simulink model "simulinkFIRDA"  (R2020b)
settings: Solver=VariableStepAuto  StartTime=0.0  StopTime=100  RelTol=1e-3
undefined symbols (not defined in the file): magnitude
libraries: simulink x3
settings Model: Creator=admin  LastModifiedBy=firda
settings SolverCC: ZeroCrossAlgorithm=Adaptive  AlgebraicLoopSolver=LineSearch
settings DataIOCC: ReturnWorkspaceOutputs=off
settings DebuggingCC: MaskedZcDiagnostic=none  IgnoredZcDiagnostic=none  ArithmeticOperatorsInVariantConditions=warning
settings SFSimCC: SimUseLocalCustomCode=off  CustomCodeUndefinedFunction=UseInterfaceOnly
settings RTWCC: RTWUseLocalCustomCode=off
settings CodeAppCC: StateflowObjectComments=on

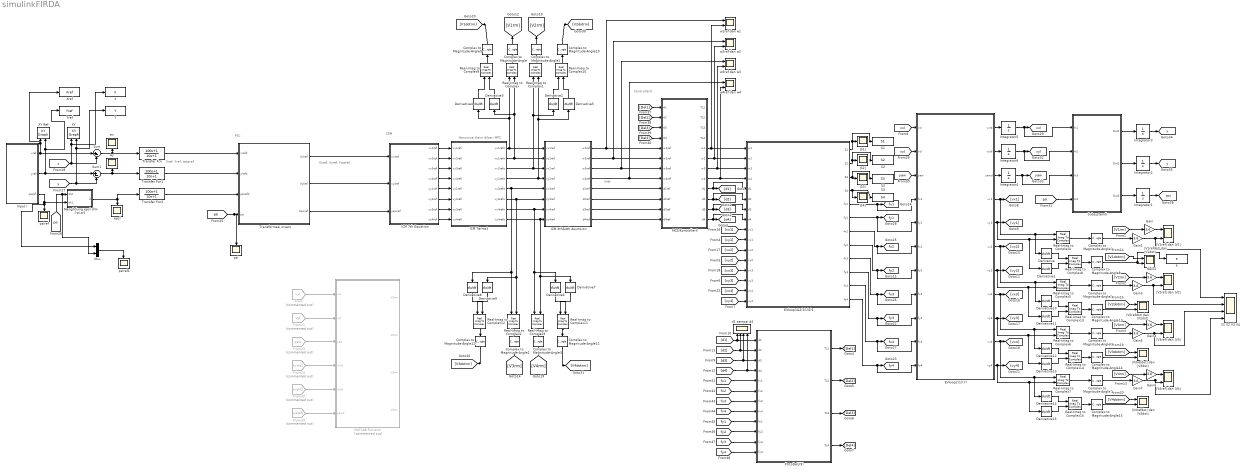
== system simulinkFIRDA ==
  note: Harusnya disini diberi MPC
  note: ControllerX
  note: C8M
  note: Xref, Yref, tetaref
  note: PTC
  note: Vxref, Vyref, Yawref
  note: Xref
  Complex to Magnitude-Angle{,1..15} (16 alike) : ComplexToMagnitudeAngle  Output=Magnitude
  Derivative{,1..15} (16 alike) : Derivative
  EVloop1&2(3)-(6)1 : Subsystem  mask(Vehicle body dinamic){re1=0.32, re2=0.32, re3=0.32, re4=0.32, m=1000, g=9.8, h=0.42, ld=0.75, lf=1.42, lr=1.42, kro=20972, kfo=50539, ksj=0.95}
      mask prompts: re1 "jari-jari roda 1 (m)"; re2 "jari-jari roda 2 (m)"; re3 "jari-jari roda 3 (m)"; re4 "jari-jari roda 4 (m)"; m "massa kendaraan (kg)"; g "percepatan gravitasi (m/s^2)"; h "tinggi pusat massa dari permukaan jalan (m)"; ld "jarak pusat massa ke bodi samping (m)"; lf "jarak pusat massa ke bodi depan (m)"; lr "jarak pusat massa ke bodi belakang (m)"; kro "ketegangan roll belakang"; kfo "ketegangan roll depan"; ksj "faktor atenuasi"
      mask help: Persamaan (3)(4)(5)(6)
  EVloop2(1)(7) : Subsystem  mask(Vehicle bodi dinamic){m=1000, ld=0.75, lf=1.42, lr=1.42, Jz=1950}
      mask prompts: m "massa kendaraan (kg)"; ld "jarak pusat massa ke bodi samping (m)"; lf "jarak pusat massa ke bodi depan (m)"; lr "jarak pusat massa ke bodi belakang (m)"; Jz "the moment of inertia of the vehicle about an axis through its CM"
      mask help: Loop 2 Persamaan 1 & 7
  From : From  Commented=on  GotoTag=vxl  TagVisibility=global
  From21 : From  Commented=on  GotoTag=vyl  TagVisibility=global
  From23 : From  Commented=on  GotoTag=yaw  TagVisibility=global
  From24 : From  Commented=on  GotoTag=vxld
  From32 : From  Commented=on  GotoTag=vyld
  From33 : From  Commented=on  GotoTag=yawd
  FtrtoDelj(9) : Subsystem  mask(Vehicle body dinamic){jm1=0.36, jm2=0.36, jm3=0.36, jm4=0.36, re1=0.32, re2=0.32, re3=0.32, re4=0.32}
      mask prompts: jm1 "momen inersia roda 1 (kgm^2)"; jm2 "momen inersia roda 2 (kgm^2)"; jm3 "momen inersia roda 3 (kgm^2)"; jm4 "momen inersia roda 4 (kgm^2)"; re1 "jari-jari roda 1 (m)"; re2 "jari-jari roda 2 (m)"; re3 "jari-jari roda 3 (m)"; re4 "jari-jari roda 4 (m)"
      mask help: Persamaan (9)
  Gain{,1..7} (8 alike) : Gain  Gain=3.6
  ICM 3th&4th Asumsion : Subsystem  mask(Persamaan ICM){rej=0.32}
      mask prompts: rej "Jari-jari roda (m)"
      mask help:
      | Asumsi 3 (Zero Slip), bidang roda berhimpit dengan Vj, aj=0,
      | djref=sudut apit (vxjref dan vyjref)
      | Asumsi 4 (Free Rolling), slip longitudinal SLj=0,
      | wjref= norm(vxjref,vyjref)/rej
  ICM 7th Equation : Subsystem  mask(Persamaan ICM){ld=0.75, lf=1.42, lr=1.42}
      mask prompts: ld "Jarak pusat masa ke bodi samping (m)"; lf "Jarak pusat masa ke bodi depan (m)"; lr "Jarak pusat masa ke bodi belakang (m)"
      mask help:
      | mengkoordinasikan kecepatan masing-masing roda
      | terhadap kecepatan pusat kendaraan
      | dengan menggunakan konsep ICM
  ICM Terms1 : Subsystem  mask(Ketentuan ICM){}
      mask help:
      | djref tidak terdefinisi ketika vxjref=vyjref=0
      | vxjref dan vyjref mengambil nilai sebelumnya saat keduanya sama dengan nol
  Input r : Subsystem  mask{Ts=0.01}
      mask prompts: Ts "Sample Period"
      mask Display: image('D:\icon mask\eight curved.jpg');
  Integrator{1..4,6} (5 alike) : Integrator
  Integrator5 : Integrator  InitialCondition=1.6
  MATLAB Function : MATLAB Function  Commented=on  TreatAsAtomicUnit=on  mask{Ts=0.01, Nc=2, Np=10, t=100, Qmat=0, Rmat=0}
      mask prompts: Ts "Sampling Time"; Nc "Control Horizon (Nc)"; Np "Prediction Horizon (Np)"; t "Run Time"; Qmat "Q"; Rmat "R"
  MCS/KontrollerX : Subsystem  mask(MCS/Kontroller X){}
      mask help: Melacak nilai torsi dan ws dari Xref
  Menghtiung epsi dlm [-pi,pi] : MATLAB Function  TreatAsAtomicUnit=on
  Mux : Mux  Inputs=2
  Real-Imag to Complex{,1..15} (16 alike) : RealImagToComplex
  S1 : ToWorkspace  VariableName=S1  SampleTime=-1
      settings: Save2DSignal=2-D array (concatenate along first dimension)
  S2 : ToWorkspace  VariableName=S2  SampleTime=-1
      settings: Save2DSignal=2-D array (concatenate along first dimension)
  S3 : ToWorkspace  VariableName=S3  SampleTime=-1
      settings: Save2DSignal=2-D array (concatenate along first dimension)
  S4 : ToWorkspace  VariableName=S4  SampleTime=-1
      settings: Save2DSignal=2-D array (concatenate along first dimension)
  Subsystem5 : Subsystem
  Sum : Sum  Inputs=|+-
  Sum1 : Sum  Inputs=|+-
  Transfer Fcn : TransferFcn  Numerator=[100 1]  Denominator=[10 1]
  Transfer Fcn1 : TransferFcn  Numerator=[100 1]  Denominator=[10 1]
  Transfer Fcn2 : TransferFcn  Numerator=[100 1]  Denominator=[10 1]
  "Transformasi invers " : Subsystem  mask(Tranformasi){}
      mask help: Mengubah Xdot menjadi Vxl Vyl Yaw
      mask Display: image('D:\icon mask\transformasi.jpg');
  V1 V2 V3 V4 : Scope  NumInputPorts=4
  X : ToWorkspace  VariableName=X  SampleTime=-1
      settings: Save2DSignal=2-D array (concatenate along first dimension)
  "XY " : simulink/Sinks/XY Graph  xmin=-40  xmax=200  ymin=-5  ymax=85  st=0.5
  XY Ref : simulink/Sinks/XY Graph  xmin=-40  xmax=200  ymin=-5  ymax=85  st=0.5
  Xref : ToWorkspace  VariableName=Xref  SampleTime=-1
      settings: Save2DSignal=2-D array (concatenate along first dimension)
  Y : ToWorkspace  VariableName=Y  SampleTime=-1
      settings: Save2DSignal=2-D array (concatenate along first dimension)
  Yref : ToWorkspace  VariableName=Yref  SampleTime=-1
      settings: Save2DSignal=2-D array (concatenate along first dimension)
  a : ToWorkspace  VariableName=a  SampleTime=-1
      settings: Save2DSignal=2-D array (concatenate along first dimension)
  d1 sampai d4 : Scope  NumInputPorts=4
  epsi : Scope
  ex : Scope
  ey : Scope
  psi : Scope
  psiref : Scope
  psiref1 : Scope
  w1ref dan w1 : Scope  NumInputPorts=2
  w2ref dan w2 : Scope  NumInputPorts=2
  w3ref dan w3 : Scope  NumInputPorts=2
  w4ref dan w4 : Scope  NumInputPorts=2
  |S1| : Scope
  |S2| : Scope
  |S3| : Scope
  |S4| : Scope
  |V1refdot| dan |V1dot| : Scope  NumInputPorts=2
  |V1ref| dan |V1| : Scope  NumInputPorts=2
  |V2refdot| dan |V2dot| : Scope  NumInputPorts=2
  |V2ref| dan |V2| : Scope  NumInputPorts=2
  |V3refdot| dan |V3dot| : Scope  NumInputPorts=2
  |V3ref| dan |V3| : Scope  NumInputPorts=2
  |V4refdot| dan |V4dot| : Scope  NumInputPorts=2
  |V4ref| dan |V4| : Scope  NumInputPorts=2
  tag scope: fx1=global, fx2=global, fx3=global, fx4=global, fy1=global, fy2=global, fy3=global, fy4=global, psi=global, vxl=global, vyl=global, x=global, y=global, yaw=global
  wires:
  [x] -> Sum/2, X/1, "XY "/1
  [y] -> Sum1/2, Y/1, "XY "/2
  [vx4] -> EVloop1&2(3)-(6)1/15(vx4)
  [vx3] -> EVloop1&2(3)-(6)1/13(vx3)
  Transfer Fcn1/1 -> "Transformasi invers "/2(yrefd)
  Transfer Fcn2/1 -> "Transformasi invers "/3(psirefd)
  "Transformasi invers "/1(Vxlref) -> ICM 7th Equation/1(vxlref)
  "Transformasi invers "/2(Vylref) -> ICM 7th Equation/2(vylref)
  "Transformasi invers "/3(Yawref) -> ICM 7th Equation/3(yawref)
  EVloop1&2(3)-(6)1/12(fy4) -> EVloop2(1)(7)/11(fy4), [fy4]
  EVloop1&2(3)-(6)1/10(fy3) -> EVloop2(1)(7)/9(fy3), [fy3]
  EVloop1&2(3)-(6)1/5(fx1) -> EVloop2(1)(7)/4(fx1), [fx1]
  EVloop1&2(3)-(6)1/7(fx2) -> EVloop2(1)(7)/6(fx2), [fx2]
  EVloop1&2(3)-(6)1/8(fy2) -> EVloop2(1)(7)/7(fy2), [fy2]
  EVloop1&2(3)-(6)1/6(fy1) -> EVloop2(1)(7)/5(fy1), [fy1]
  [vy4] -> EVloop1&2(3)-(6)1/16(vy4)
  [vy3] -> EVloop1&2(3)-(6)1/14(vy3)
  [vy2] -> EVloop1&2(3)-(6)1/12(vy2)
  [vx2] -> EVloop1&2(3)-(6)1/11(vx2)
  [vy1] -> EVloop1&2(3)-(6)1/10(vy1)
  [vx1] -> EVloop1&2(3)-(6)1/9(vx1)
  [Del1] -> MCS/KontrollerX/1(tl1)
  [Del2] -> MCS/KontrollerX/2(tl2)
  ICM 3th&4th Asumsion/1(w1ref) -> MCS/KontrollerX/5(w1ref), w1ref dan w1/1
  ICM 3th&4th Asumsion/5(d1ref) -> MCS/KontrollerX/9(d1ref)
  ICM 3th&4th Asumsion/2(w2ref) -> MCS/KontrollerX/6(w2ref), w2ref dan w2/1
  [Del3] -> MCS/KontrollerX/3(tl3)
  ICM 3th&4th Asumsion/6(d2ref) -> MCS/KontrollerX/10(d2ref)
  ICM 3th&4th Asumsion/3(w3ref) -> MCS/KontrollerX/7(w3ref), w3ref dan w3/1
  ICM 3th&4th Asumsion/7(d3ref) -> MCS/KontrollerX/11(d3ref)
  [Del4] -> MCS/KontrollerX/4(tl4)
  ICM 3th&4th Asumsion/4(w4ref) -> MCS/KontrollerX/8(w4ref), w4ref dan w4/1
  ICM 3th&4th Asumsion/8(d4ref) -> MCS/KontrollerX/12(d4ref)
  Integrator3/1 -> [x]
  Integrator2/1 -> [y]
  Integrator1/1 -> [psi]
  EVloop1&2(3)-(6)1/9(fx3) -> EVloop2(1)(7)/8(fx3), [fx3]
  EVloop1&2(3)-(6)1/11(fx4) -> EVloop2(1)(7)/10(fx4), [fx4]
  [vxl] -> EVloop2(1)(7)/1(vxl)
  [vyl] -> EVloop2(1)(7)/2(vyl)
  [yaw] -> EVloop2(1)(7)/3(yaw)
  EVloop2(1)(7)/4(vx1) -> Derivative/1, Real-Imag to Complex4/1, [vx1]
  EVloop2(1)(7)/5(vy1) -> Derivative1/1, Real-Imag to Complex4/2, [vy1]
  EVloop2(1)(7)/1(vxld) -> Integrator5/1
  Integrator5/1 -> Subsystem5/1(In1), [vxl]
  EVloop2(1)(7)/2(vyld) -> Integrator6/1
  Integrator6/1 -> Subsystem5/2(In2), [vyl]
  EVloop2(1)(7)/3(yawd) -> Integrator4/1
  Integrator4/1 -> Subsystem5/3(In3), [yaw]
  [psi] -> Subsystem5/4(In4)
  Subsystem5/1(Out1) -> Integrator3/1
  Subsystem5/2(Out2) -> Integrator2/1
  Subsystem5/3(Out3) -> Integrator1/1
  MCS/KontrollerX/9(d1) -> EVloop1&2(3)-(6)1/5(d1), [d1]
  MCS/KontrollerX/10(d2) -> EVloop1&2(3)-(6)1/6(d2), [d2]
  MCS/KontrollerX/11(d3) -> EVloop1&2(3)-(6)1/7(d3), [d3]
  MCS/KontrollerX/12(d4) -> EVloop1&2(3)-(6)1/8(d4), [d4]
  MCS/KontrollerX/5(w1) -> EVloop1&2(3)-(6)1/1(w1), w1ref dan w1/2
  MCS/KontrollerX/6(w2) -> EVloop1&2(3)-(6)1/2(w2), w2ref dan w2/2
  MCS/KontrollerX/7(w3) -> EVloop1&2(3)-(6)1/3(w3), w3ref dan w3/2
  MCS/KontrollerX/8(w4) -> EVloop1&2(3)-(6)1/4(w4), w4ref dan w4/2
  Transfer Fcn/1 -> "Transformasi invers "/1(xrefd)
  ICM 7th Equation/1(vx1ref) -> ICM Terms1/1(vx1refi)
  ICM 7th Equation/2(vx2ref) -> ICM Terms1/2(vx2refi)
  ICM 7th Equation/3(vx3ref) -> ICM Terms1/3(vx3refi)
  ICM 7th Equation/4(vx4ref) -> ICM Terms1/4(vx4refi)
  ICM 7th Equation/5(vy1ref) -> ICM Terms1/5(vy1refi)
  ICM 7th Equation/6(vy2ref) -> ICM Terms1/6(vy2refi)
  ICM 7th Equation/7(vy3ref) -> ICM Terms1/7(vy3refi)
  ICM 7th Equation/8(vy4ref) -> ICM Terms1/8(vy4refi)
  ICM Terms1/1(vx1refo) -> ICM 3th&4th Asumsion/1(vx1ref), Derivative4/1, Real-Imag to Complex/1
  ICM Terms1/2(vy1refo) -> ICM 3th&4th Asumsion/2(vy1ref), Derivative3/1, Real-Imag to Complex/2
  ICM Terms1/3(vx2refo) -> Real-Imag to Complex1/1, Derivative2/1, ICM 3th&4th Asumsion/3(vx2ref)
  ICM Terms1/4(vy2refo) -> Derivative5/1, Real-Imag to Complex1/2, ICM 3th&4th Asumsion/4(vy2ref)
  Sum/1 -> Transfer Fcn/1, ex/1
  Sum1/1 -> ey/1, Transfer Fcn1/1
  Input r/1(xref) -> Sum/1, Xref/1, XY Ref/1
  EVloop1&2(3)-(6)1/1(S1) -> S1/1, |S1|/1
  Input r/2(yref) -> Sum1/1, Yref/1, XY Ref/2
  EVloop1&2(3)-(6)1/2(S2) -> S2/1, |S2|/1
  EVloop1&2(3)-(6)1/3(S3) -> |S3|/1, S3/1
  EVloop1&2(3)-(6)1/4(S4) -> |S4|/1, S4/1
  [fy3] -> FtrtoDelj(9)/11(fy3)
  [fy1] -> FtrtoDelj(9)/9(fy1)
  [d1] -> FtrtoDelj(9)/1(d1), d1 sampai d4/1
  FtrtoDelj(9)/3(TL3) -> [Del3]
  [fy2] -> FtrtoDelj(9)/10(fy2)
  FtrtoDelj(9)/1(TL1) -> [Del1]
  FtrtoDelj(9)/2(TL2) -> [Del2]
  [d3] -> FtrtoDelj(9)/3(d3), d1 sampai d4/3
  [d4] -> d1 sampai d4/4, FtrtoDelj(9)/4(d4)
  [fx4] -> FtrtoDelj(9)/8(fx4)
  [fx1] -> FtrtoDelj(9)/5(fx1)
  [fx3] -> FtrtoDelj(9)/7(fx3)
  [d2] -> FtrtoDelj(9)/2(d2), d1 sampai d4/2
  [fx2] -> FtrtoDelj(9)/6(fx2)
  [fy4] -> FtrtoDelj(9)/12(fy4)
  FtrtoDelj(9)/4(TL4) -> [Del4]
  Real-Imag to Complex/1 -> Complex to Magnitude-Angle/1
  Complex to Magnitude-Angle/1 -> [V1rm]
  Real-Imag to Complex1/1 -> Complex to Magnitude-Angle1/1
  Complex to Magnitude-Angle1/1 -> [V2rm]
  Real-Imag to Complex2/1 -> Complex to Magnitude-Angle2/1
  Complex to Magnitude-Angle2/1 -> [V3rm]
  Complex to Magnitude-Angle3/1 -> [V4rm]
  Real-Imag to Complex3/1 -> Complex to Magnitude-Angle3/1
  Real-Imag to Complex4/1 -> Complex to Magnitude-Angle4/1
  Complex to Magnitude-Angle4/1 -> Gain1/1
  Real-Imag to Complex5/1 -> Complex to Magnitude-Angle5/1
  Complex to Magnitude-Angle5/1 -> Gain3/1
  [V2rm] -> Gain2/1
  Real-Imag to Complex6/1 -> Complex to Magnitude-Angle6/1
  Complex to Magnitude-Angle6/1 -> Gain5/1
  [V3rm] -> Gain4/1
  Real-Imag to Complex7/1 -> Complex to Magnitude-Angle7/1
  [V4rm] -> Gain6/1
  [psi] -> psi/1, "Transformasi invers "/4(psi)
  Input r/3("psiref ") -> Menghtiung epsi dlm [-pi,pi]/2(th1), Mux/1, psiref/1
  [psi] -> Mux/2, Menghtiung epsi dlm [-pi,pi]/1(th2)
  Menghtiung epsi dlm [-pi,pi]/1(d) -> Transfer Fcn2/1, epsi/1
  Derivative/1 -> Real-Imag to Complex8/1
  Derivative1/1 -> Real-Imag to Complex8/2
  Real-Imag to Complex8/1 -> Complex to Magnitude-Angle8/1
  Derivative3/1 -> Real-Imag to Complex9/2
  Derivative4/1 -> Real-Imag to Complex9/1
  Complex to Magnitude-Angle9/1 -> [V1dotrm]
  Real-Imag to Complex9/1 -> Complex to Magnitude-Angle9/1
  Complex to Magnitude-Angle10/1 -> [V2dotrm]
  Derivative5/1 -> Real-Imag to Complex10/2
  Derivative2/1 -> Real-Imag to Complex10/1
  Real-Imag to Complex10/1 -> Complex to Magnitude-Angle10/1
  Complex to Magnitude-Angle11/1 -> [V4dotrm]
  Derivative6/1 -> Real-Imag to Complex11/2
  ICM Terms1/7(vx4refo) -> ICM 3th&4th Asumsion/7(vx4ref), Derivative6/1, Real-Imag to Complex3/1
  ICM Terms1/8(vy4refo) -> ICM 3th&4th Asumsion/8(vy4ref), Derivative7/1, Real-Imag to Complex3/2
  Derivative7/1 -> Real-Imag to Complex11/1
  Real-Imag to Complex11/1 -> Complex to Magnitude-Angle11/1
  Complex to Magnitude-Angle12/1 -> [V3dotrm]
  Derivative8/1 -> Real-Imag to Complex12/2
  ICM Terms1/5(vx3refo) -> ICM 3th&4th Asumsion/5(vx3ref), Real-Imag to Complex2/1, Derivative8/1
  ICM Terms1/6(vy3refo) -> ICM 3th&4th Asumsion/6(vy3ref), Real-Imag to Complex2/2, Derivative9/1
  Derivative9/1 -> Real-Imag to Complex12/1
  Real-Imag to Complex12/1 -> Complex to Magnitude-Angle12/1
  [V2dotrm] -> |V2refdot| dan |V2dot|/1
  EVloop2(1)(7)/7(vy2) -> Derivative11/1, Real-Imag to Complex5/2, [vy2]
  Derivative10/1 -> Real-Imag to Complex13/1
  Complex to Magnitude-Angle13/1 -> |V2refdot| dan |V2dot|/2
  Real-Imag to Complex13/1 -> Complex to Magnitude-Angle13/1
  Derivative11/1 -> Real-Imag to Complex13/2
  EVloop2(1)(7)/6(vx2) -> Derivative10/1, Real-Imag to Complex5/1, [vx2]
  [V3dotrm] -> |V3refdot| dan |V3dot|/1
  EVloop2(1)(7)/9(vy3) -> Derivative13/1, Real-Imag to Complex6/2, [vy3]
  Derivative12/1 -> Real-Imag to Complex14/1
  Complex to Magnitude-Angle14/1 -> |V3refdot| dan |V3dot|/2
  Real-Imag to Complex14/1 -> Complex to Magnitude-Angle14/1
  Derivative13/1 -> Real-Imag to Complex14/2
  EVloop2(1)(7)/8(vx3) -> Derivative12/1, Real-Imag to Complex6/1, [vx3]
  [V4dotrm] -> |V4refdot| dan |V4dot|/1
  EVloop2(1)(7)/11(vy4) -> Derivative15/1, Real-Imag to Complex7/2, [vy4]
  Derivative14/1 -> Real-Imag to Complex15/1
  Complex to Magnitude-Angle15/1 -> |V4refdot| dan |V4dot|/2
  Real-Imag to Complex15/1 -> Complex to Magnitude-Angle15/1
  Derivative15/1 -> Real-Imag to Complex15/2
  EVloop2(1)(7)/10(vx4) -> Derivative14/1, Real-Imag to Complex7/1, [vx4]
  Complex to Magnitude-Angle7/1 -> Gain7/1
  [V1rm] -> Gain/1
  Gain/1 -> |V1ref| dan |V1|/1
  Gain1/1 -> V1 V2 V3 V4/1, |V1ref| dan |V1|/2
  Gain2/1 -> |V2ref| dan |V2|/1
  Gain3/1 -> V1 V2 V3 V4/2, |V2ref| dan |V2|/2
  Gain4/1 -> |V3ref| dan |V3|/1
  Gain5/1 -> |V3ref| dan |V3|/2, V1 V2 V3 V4/3
  Gain6/1 -> |V4ref| dan |V4|/1
  Gain7/1 -> V1 V2 V3 V4/4, |V4ref| dan |V4|/2
  Complex to Magnitude-Angle8/1 -> a/1, |V1refdot| dan |V1dot|/2
  Mux/1 -> psiref1/1
  From/1 -> MATLAB Function/1(vxl)
  From21/1 -> MATLAB Function/2(vyl)
  From23/1 -> MATLAB Function/3(yaw)
  From33/1 -> MATLAB Function/6(yawd)
  From32/1 -> MATLAB Function/5(vyld)
  From24/1 -> MATLAB Function/4(vxld)
  [V1dotrm] -> |V1refdot| dan |V1dot|/1

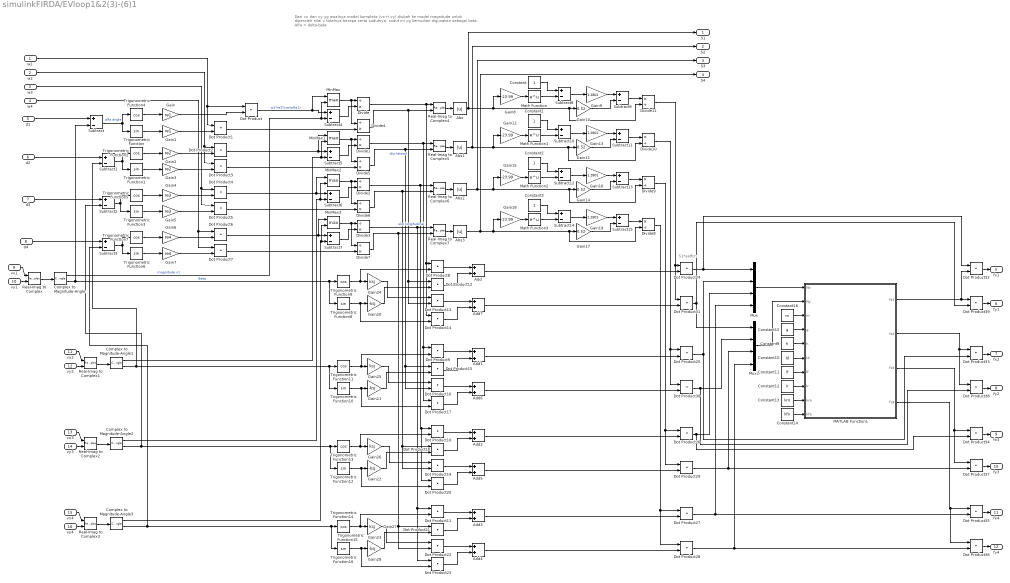
== system simulinkFIRDA/EVloop1&2(3)-(6)1 ==
  note: S1*satfcn
  note: Dari vx dan vy yg awalnya model kompleks (vx+i vy) diubah ke model magnitude untuk diperoleh nilai v totalnya berapa serta sudutnya. sudut ini yg kemudian digunakan sebagai beta.
      | Alfa = delta-beta
  w1 : Inport
  w2 : Inport  Port=2
  w3 : Inport  Port=3
  w4 : Inport  Port=4
  d1 : Inport  Port=5
  d2 : Inport  Port=6
  d3 : Inport  Port=7
  d4 : Inport  Port=8
  vx1 : Inport  Port=9
  vy1 : Inport  Port=10
  vx2 : Inport  Port=11
  vy2 : Inport  Port=12
  vx3 : Inport  Port=13
  vy3 : Inport  Port=14
  vx4 : Inport  Port=15
  vy4 : Inport  Port=16
  Abs{,1..3} (4 alike) : Abs
  Add{,1..7} (8 alike) : Sum
  Complex to Magnitude-Angle{,1..3} (4 alike) : ComplexToMagnitudeAngle
  Constant{,1..3} (4 alike) : Constant
  Constant10 : Constant  Value=ld
  Constant11 : Constant  Value=lf
  Constant12 : Constant  Value=lr
  Constant13 : Constant  Value=kro
  Constant14 : Constant  Value=kfo
  Constant15 : Constant  Value=g
  Constant16 : Constant  Value=m
  Constant9 : Constant  Value=h
  Divide{,1..7} (8 alike) : Product  Inputs=/*
  Divide{8..11} (4 alike) : Product  Inputs=*/
  Dot Product{,1..39} (40 alike) : DotProduct  InputSameDT=on  OutDataTypeStr=Inherit: Inherit via internal rule
  Gain : Gain  Gain=re1
  Gain1 : Gain  Gain=re1
  Gain{10..11,14,17} (4 alike) : Gain  Gain=0.52
  Gain{8,12,15,18} (4 alike) : Gain  Gain=-23.99
  Gain{9,13,16,19} (4 alike) : Gain  Gain=1.2801
  Gain2 : Gain  Gain=re2
  Gain{20..23,28} (5 alike) : Gain  Gain=-ksj
  Gain{24..27} (4 alike) : Gain  Gain=ksj
  Gain3 : Gain  Gain=re2
  Gain4 : Gain  Gain=re3
  Gain5 : Gain  Gain=re3
  Gain6 : Gain  Gain=re4
  Gain7 : Gain  Gain=re4
  MATLAB Function1 : MATLAB Function  TreatAsAtomicUnit=on
  Math Function{,1..3} (4 alike) : Math  SignedPower=on  SaturateOnIntegerOverflow=on
  MinMax{,1..3} (4 alike) : MinMax  Function=max  Inputs=2
  Mux : Mux
  Mux1 : Mux
  Real-Imag to Complex{,1..7} (8 alike) : RealImagToComplex
  Subtract{,1..15} (16 alike) : Sum  Inputs=+-
  Trigonometric Function{,1,3,6,8,10,12,14,16} (9 alike) : Trigonometry
  Trigonometric Function{2,4..5,7,9,11,13,15} (8 alike) : Trigonometry  Operator=cos
  S1 : Outport
  S2 : Outport  Port=2
  S3 : Outport  Port=3
  S4 : Outport  Port=4
  fx1 : Outport  Port=5
  fy1 : Outport  Port=6
  fx2 : Outport  Port=7
  fy2 : Outport  Port=8
  fx3 : Outport  Port=9
  fy3 : Outport  Port=10
  fx4 : Outport  Port=11
  fy4 : Outport  Port=12
  wires:
  Dot Product33/1 -> fx2/1
  Dot Product35/1 -> fx4/1
  Dot Product28/1 -> Dot Product36/2, Mux1/4
  Dot Product36/1 -> fy4/1
  Dot Product34/1 -> fx3/1
  Dot Product39/1 -> fy1/1
  Dot Product37/1 -> fy3/1
  Dot Product38/1 -> fy2/1
  Dot Product32/1 -> fx1/1
  vx1/1 -> Real-Imag to Complex/1
  vy1/1 -> Real-Imag to Complex/2
  vx3/1 -> Real-Imag to Complex2/1
  vy3/1 -> Real-Imag to Complex2/2
  vx4/1 -> Real-Imag to Complex3/1
  vx2/1 -> Real-Imag to Complex1/1
  vy4/1 -> Real-Imag to Complex3/2
  vy2/1 -> Real-Imag to Complex1/2
  Constant15/1 -> MATLAB Function1/4(g)
  Dot Product31/1 -> Dot Product39/2, Mux1/1
  Dot Product29/1 -> Dot Product37/2, Mux1/3
  Dot Product30/1 -> Dot Product38/2, Mux1/2
  Constant16/1 -> MATLAB Function1/3(m)
  MATLAB Function1/1(fz1) -> Dot Product32/2, Dot Product39/1
  MATLAB Function1/3(fz3) -> Dot Product34/1, Dot Product37/1
  Constant14/1 -> MATLAB Function1/10(kfo)
  Constant13/1 -> MATLAB Function1/9(kro)
  Real-Imag to Complex2/1 -> Complex to Magnitude-Angle2/1
  Real-Imag to Complex3/1 -> Complex to Magnitude-Angle3/1
  Complex to Magnitude-Angle/2 -> Trigonometric Function8/1, Trigonometric Function9/1, Subtract/2  "Beta"
  Complex to Magnitude-Angle1/2 -> Trigonometric Function10/1, Trigonometric Function11/1, Subtract1/2
  Real-Imag to Complex/1 -> Complex to Magnitude-Angle/1
  Real-Imag to Complex1/1 -> Complex to Magnitude-Angle1/1
  Trigonometric Function1/1 -> Gain3/1
  w1/1 -> Dot Product1/1, Dot Product/1
  Trigonometric Function5/1 -> Gain4/1
  d4/1 -> Subtract3/1
  Subtract/1 -> Trigonometric Function/1, Trigonometric Function4/1  "alfa angle"
  Gain4/1 -> Dot Product4/2
  w2/1 -> Dot Product2/1, Dot Product3/1
  w4/1 -> Dot Product6/1, Dot Product7/1
  Subtract2/1 -> Trigonometric Function3/1, Trigonometric Function5/1
  d3/1 -> Subtract2/1
  Gain5/1 -> Dot Product5/2
  Gain/1 -> Dot Product/2
  Dot Product2/1 -> MinMax1/1, Subtract5/1
  Gain1/1 -> Dot Product1/2
  d1/1 -> Subtract/1
  Gain3/1 -> Dot Product3/2
  Gain7/1 -> Dot Product7/2
  Trigonometric Function6/1 -> Gain7/1
  Dot Product/1 -> Subtract4/1, MinMax/1  "w1*re1*cos(alfa1)"
  Complex to Magnitude-Angle3/2 -> Subtract3/2, Trigonometric Function16/1, Trigonometric Function14/1, Trigonometric Function15/1
  Trigonometric Function4/1 -> Gain/1
  Complex to Magnitude-Angle2/2 -> Trigonometric Function12/1, Trigonometric Function13/1, Subtract2/2
  Subtract1/1 -> Trigonometric Function2/1, Trigonometric Function1/1
  Trigonometric Function2/1 -> Gain2/1
  Trigonometric Function3/1 -> Gain5/1
  Gain6/1 -> Dot Product6/2
  Trigonometric Function/1 -> Gain1/1
  Gain2/1 -> Dot Product2/2
  w3/1 -> Dot Product4/1, Dot Product5/1
  Trigonometric Function7/1 -> Gain6/1
  d2/1 -> Subtract1/1
  Subtract3/1 -> Trigonometric Function6/1, Trigonometric Function7/1
  Complex to Magnitude-Angle/1 -> MinMax/2, Subtract4/2  "magnitude v1"
  Real-Imag to Complex5/1 -> Abs1/1
  Divide3/1 -> Dot Product23/1, Dot Product11/1, Real-Imag to Complex7/1
  Dot Product5/1 -> Divide6/2
  Divide/1 -> Dot Product14/1, Dot Product8/1, Real-Imag to Complex4/1  "slip longitudinal"
  Real-Imag to Complex6/1 -> Abs2/1
  MinMax3/1 -> Divide7/1, Divide3/1
  Divide7/1 -> Dot Product22/2, Dot Product21/1, Real-Imag to Complex7/2
  MinMax1/1 -> Divide5/1, Divide1/1
  Dot Product3/1 -> Divide5/2
  Dot Product7/1 -> Divide7/2
  Subtract5/1 -> Divide1/2
  Divide6/1 -> Dot Product19/2, Dot Product18/1, Real-Imag to Complex6/2
  Real-Imag to Complex7/1 -> Abs3/1
  Complex to Magnitude-Angle3/1 -> MinMax3/2, Subtract7/2
  Dot Product4/1 -> MinMax2/1, Subtract6/1
  Dot Product6/1 -> MinMax3/1, Subtract7/1
  Real-Imag to Complex4/1 -> Abs/1
  Gain8/1 -> Math Function/1
  Subtract6/1 -> Divide2/2
  Math Function/1 -> Subtract8/2
  Divide4/1 -> Dot Product13/2, Dot Product12/1, Real-Imag to Complex4/2  "slip lateral"
  Complex to Magnitude-Angle2/1 -> MinMax2/2, Subtract6/2
  Dot Product1/1 -> Divide4/2
  Subtract4/1 -> Divide/2
  Complex to Magnitude-Angle1/1 -> MinMax1/2, Subtract5/2
  MinMax/1 -> Divide4/1, Divide/1
  Subtract7/1 -> Divide3/2
  Divide5/1 -> Dot Product15/1, Dot Product16/2, Real-Imag to Complex5/2
  Divide2/1 -> Dot Product20/1, Dot Product10/1, Real-Imag to Complex6/1
  MinMax2/1 -> Divide6/1, Divide2/1
  Divide1/1 -> Dot Product9/1, Dot Product17/1, Real-Imag to Complex5/1
  Gain9/1 -> Subtract9/1
  Gain12/1 -> Math Function1/1
  Trigonometric Function8/1 -> Dot Product14/2, Gain20/1
  Trigonometric Function10/1 -> Dot Product17/2, Gain21/1
  Gain10/1 -> Subtract9/2
  Subtract8/1 -> Gain9/1
  Trigonometric Function14/1 -> Gain23/1
  Subtract14/1 -> Gain19/1
  Abs3/1 -> S4/1, Gain18/1, Gain17/1, Divide8/2
  Abs2/1 -> S3/1, Gain15/1, Divide9/2, Gain14/1
  Subtract13/1 -> Divide9/1
  Subtract10/1 -> Gain13/1
  Gain18/1 -> Math Function3/1
  Subtract15/1 -> Divide8/1
  Constant2/1 -> Subtract12/1
  Constant1/1 -> Subtract10/1
  Constant3/1 -> Subtract14/1
  Trigonometric Function12/1 -> Dot Product20/2, Gain22/1
  Abs1/1 -> S2/1, Gain12/1, Divide10/2, Gain11/1
  Trigonometric Function9/1 -> Dot Product8/2, Gain24/1
  Gain16/1 -> Subtract13/1
  Gain17/1 -> Subtract15/2
  Constant/1 -> Subtract8/1
  Math Function1/1 -> Subtract10/2
  Gain13/1 -> Subtract11/1
  Math Function2/1 -> Subtract12/2
  Subtract12/1 -> Gain16/1
  Gain15/1 -> Math Function2/1
  Gain14/1 -> Subtract13/2
  Math Function3/1 -> Subtract14/2
  Gain19/1 -> Subtract15/1
  Gain11/1 -> Subtract11/2
  Divide9/1 -> Dot Product26/1, Dot Product29/1
  Dot Product11/1 -> Add3/1
  Trigonometric Function13/1 -> Dot Product10/2, Gain26/1
  Add3/1 -> Dot Product27/2
  Dot Product10/1 -> Add2/1
  Add2/1 -> Dot Product26/2
  Dot Product21/1 -> Add3/2
  Divide8/1 -> Dot Product28/1, Dot Product27/1
  Trigonometric Function16/1 -> Dot Product23/2, Gain28/1
  Gain24/1 -> Dot Product13/1
  Dot Product9/1 -> Add1/1
  Gain25/1 -> Dot Product16/1
  Gain26/1 -> Dot Product19/1
  Gain27/1 -> Dot Product22/1
  Add4/1 -> Dot Product28/2
  Divide11/1 -> Dot Product31/1, Dot Product24/1
  Dot Product18/1 -> Add2/2
  Add/1 -> Dot Product24/2
  Gain20/1 -> Dot Product12/2
  Dot Product8/1 -> Add/1
  Gain21/1 -> Dot Product15/2
  Gain22/1 -> Dot Product18/2
  Dot Product15/1 -> Add1/2
  Divide10/1 -> Dot Product30/1, Dot Product25/1
  Abs/1 -> S1/1, Gain8/1, Divide11/2, Gain10/1
  Trigonometric Function11/1 -> Dot Product9/2, Gain25/1
  Gain28/1 -> Dot Product21/2
  Trigonometric Function15/1 -> Dot Product11/2, Gain27/1
  Subtract9/1 -> Divide11/1
  Add1/1 -> Dot Product25/2
  Dot Product12/1 -> Add/2
  Subtract11/1 -> Divide10/1
  Add7/1 -> Dot Product31/2
  Dot Product22/1 -> Add4/1
  Dot Product16/1 -> Add6/1
  Add5/1 -> Dot Product29/2
  Dot Product17/1 -> Add6/2
  Dot Product13/1 -> Add7/1
  Dot Product19/1 -> Add5/1
  Dot Product14/1 -> Add7/2
  Add6/1 -> Dot Product30/2
  Dot Product23/1 -> Add4/2
  Dot Product20/1 -> Add5/2
  Dot Product27/1 -> Dot Product35/2, Mux/4
  Constant11/1 -> MATLAB Function1/7(lf)
  Dot Product25/1 -> Dot Product33/2, Mux/2
  Constant9/1 -> MATLAB Function1/5(h)
  Dot Product24/1 -> Dot Product32/1, Mux/1
  Constant10/1 -> MATLAB Function1/6(ld)
  Mux1/1 -> MATLAB Function1/2(Ny)
  Constant12/1 -> MATLAB Function1/8(lr)
  MATLAB Function1/4(fz4) -> Dot Product36/1, Dot Product35/1
  MATLAB Function1/2(fz2) -> Dot Product33/1, Dot Product38/1
  Dot Product26/1 -> Dot Product34/2, Mux/3
  Mux/1 -> MATLAB Function1/1(Nx)

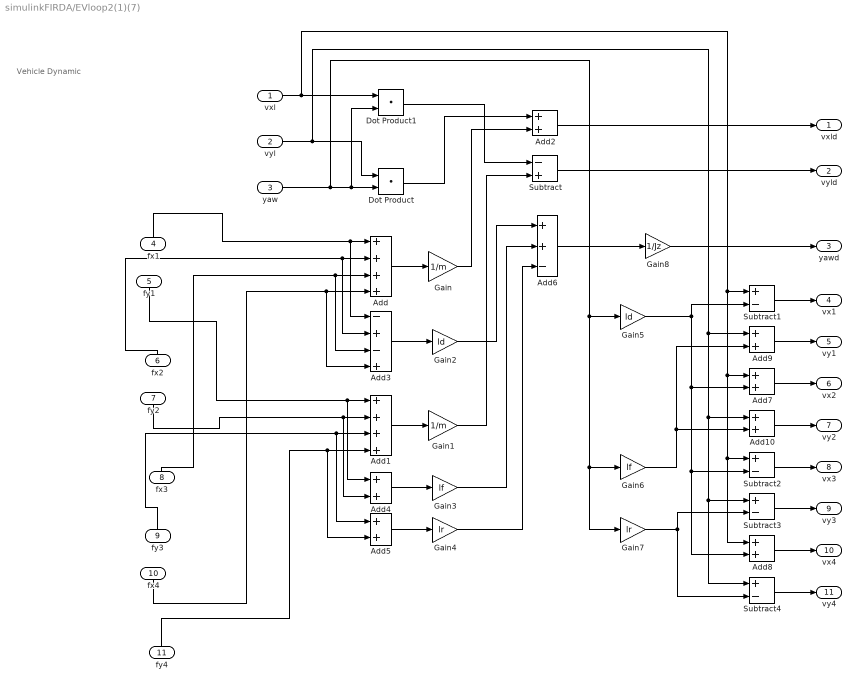
== system simulinkFIRDA/EVloop2(1)(7) ==
  note: Vehicle Dynamic
  vxl : Inport
  vyl : Inport  Port=2
  yaw : Inport  Port=3
  fx1 : Inport  Port=4
  fy1 : Inport  Port=5
  fx2 : Inport  Port=6
  fy2 : Inport  Port=7
  fx3 : Inport  Port=8
  fy3 : Inport  Port=9
  fx4 : Inport  Port=10
  fy4 : Inport  Port=11
  Add : Sum  Inputs=++++
  Add1 : Sum  Inputs=++++
  Add{2,4..5,7..10} (7 alike) : Sum
  Add3 : Sum  Inputs=-+-+
  Add6 : Sum  Inputs=++-
  Dot Product : DotProduct  InputSameDT=on  OutDataTypeStr=Inherit: Inherit via internal rule
  Dot Product1 : DotProduct  InputSameDT=on  OutDataTypeStr=Inherit: Inherit via internal rule
  Gain : Gain  Gain=1/m
  Gain1 : Gain  Gain=1/m
  Gain2 : Gain  Gain=ld
  Gain3 : Gain  Gain=lf
  Gain4 : Gain  Gain=lr
  Gain5 : Gain  Gain=ld
  Gain6 : Gain  Gain=lf
  Gain7 : Gain  Gain=lr
  Gain8 : Gain  Gain=1/Jz
  Subtract : Sum  Inputs=-+
  Subtract{1..4} (4 alike) : Sum  Inputs=+-
  vxld : Outport
  vyld : Outport  Port=2
  yawd : Outport  Port=3
  vx1 : Outport  Port=4
  vy1 : Outport  Port=5
  vx2 : Outport  Port=6
  vy2 : Outport  Port=7
  vx3 : Outport  Port=8
  vy3 : Outport  Port=9
  vx4 : Outport  Port=10
  vy4 : Outport  Port=11
  wires:
  Subtract3/1 -> vy3/1
  Add3/1 -> Gain2/1
  Add1/1 -> Gain1/1
  vxl/1 -> Add7/1, Subtract2/1, Add8/1, Subtract1/1, Dot Product1/1
  yaw/1 -> Gain7/1, Gain6/1, Gain5/1, Dot Product1/2, Dot Product/2
  Add8/1 -> vx4/1
  Add/1 -> Gain/1
  Gain6/1 -> Add10/2, Add9/2
  Gain1/1 -> Subtract/2
  vyl/1 -> Dot Product/1, Subtract4/1, Subtract3/1, Add10/1, Add9/1
  Add9/1 -> vy1/1
  Gain2/1 -> Add6/1
  Add4/1 -> Gain3/1
  Subtract4/1 -> vy4/1
  Subtract1/1 -> vx1/1
  Add6/1 -> Gain8/1
  Add10/1 -> vy2/1
  Dot Product/1 -> Add2/1
  Gain7/1 -> Subtract4/2, Subtract3/2
  Gain5/1 -> Add8/2, Subtract2/2, Add7/2, Subtract1/2
  Subtract2/1 -> vx3/1
  Subtract/1 -> vyld/1
  Dot Product1/1 -> Subtract/1
  Add7/1 -> vx2/1
  Add5/1 -> Gain4/1
  Gain3/1 -> Add6/2
  Add2/1 -> vxld/1
  Gain/1 -> Add2/2
  fy4/1 -> Add5/2, Add1/4
  fy2/1 -> Add4/2, Add1/2
  fy3/1 -> Add5/1, Add1/3
  fy1/1 -> Add1/1, Add4/1
  fx4/1 -> Add3/4, Add/4
  fx2/1 -> Add3/2, Add/2
  fx3/1 -> Add3/3, Add/3
  fx1/1 -> Add3/1, Add/1
  Gain4/1 -> Add6/3
  Gain8/1 -> yawd/1

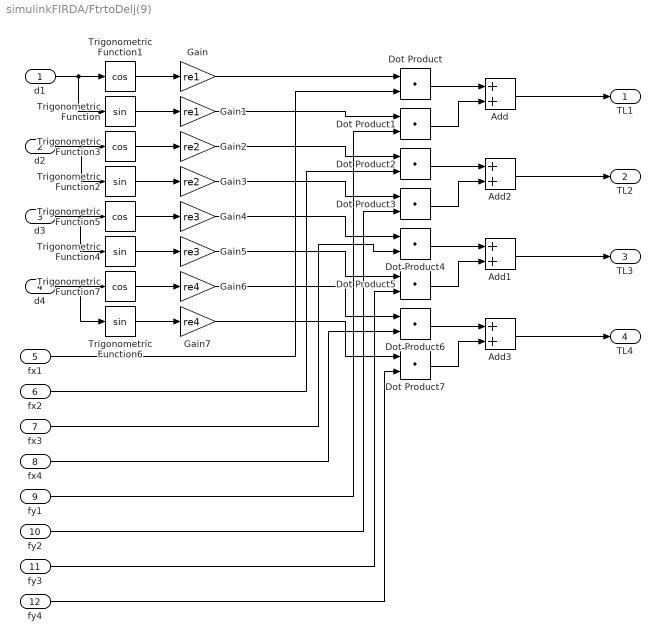
== system simulinkFIRDA/FtrtoDelj(9) ==
  d1 : Inport
  d2 : Inport  Port=2
  d3 : Inport  Port=3
  d4 : Inport  Port=4
  fx1 : Inport  Port=5
  fx2 : Inport  Port=6
  fx3 : Inport  Port=7
  fx4 : Inport  Port=8
  fy1 : Inport  Port=9
  fy2 : Inport  Port=10
  fy3 : Inport  Port=11
  fy4 : Inport  Port=12
  Add{,1..3} (4 alike) : Sum
  Dot Product{,1..7} (8 alike) : DotProduct  InputSameDT=on  OutDataTypeStr=Inherit: Inherit via internal rule
  Gain : Gain  Gain=re1
  Gain1 : Gain  Gain=re1
  Gain2 : Gain  Gain=re2
  Gain3 : Gain  Gain=re2
  Gain4 : Gain  Gain=re3
  Gain5 : Gain  Gain=re3
  Gain6 : Gain  Gain=re4
  Gain7 : Gain  Gain=re4
  Trigonometric Function{,2,4,6} (4 alike) : Trigonometry
  Trigonometric Function{1,3,5,7} (4 alike) : Trigonometry  Operator=cos
  TL1 : Outport
  TL2 : Outport  Port=2
  TL3 : Outport  Port=3
  TL4 : Outport  Port=4
  wires:
  Gain3/1 -> Dot Product3/1
  fy2/1 -> Dot Product3/2
  Dot Product2/1 -> Add2/1
  fx2/1 -> Dot Product2/2
  Add1/1 -> TL3/1
  Gain2/1 -> Dot Product2/1
  fx1/1 -> Dot Product/2
  d3/1 -> Trigonometric Function4/1, Trigonometric Function5/1
  Trigonometric Function4/1 -> Gain5/1
  Dot Product1/1 -> Add/2
  fy1/1 -> Dot Product1/2
  Dot Product5/1 -> Add1/2
  Dot Product7/1 -> Add3/2
  Add2/1 -> TL2/1
  Dot Product/1 -> Add/1
  Gain6/1 -> Dot Product6/1
  Gain5/1 -> Dot Product5/1
  d2/1 -> Trigonometric Function2/1, Trigonometric Function3/1
  Gain1/1 -> Dot Product1/1
  fx4/1 -> Dot Product6/2
  d1/1 -> Trigonometric Function/1, Trigonometric Function1/1
  fy4/1 -> Dot Product7/2
  Dot Product3/1 -> Add2/2
  Trigonometric Function2/1 -> Gain3/1
  Trigonometric Function6/1 -> Gain7/1
  Dot Product6/1 -> Add3/1
  Trigonometric Function1/1 -> Gain/1
  Add/1 -> TL1/1
  Add3/1 -> TL4/1
  fx3/1 -> Dot Product4/2
  Trigonometric Function7/1 -> Gain6/1
  Trigonometric Function3/1 -> Gain2/1
  Trigonometric Function/1 -> Gain1/1
  Gain4/1 -> Dot Product4/1
  d4/1 -> Trigonometric Function6/1, Trigonometric Function7/1
  Gain/1 -> Dot Product/1
  Trigonometric Function5/1 -> Gain4/1
  Gain7/1 -> Dot Product7/1
  Dot Product4/1 -> Add1/1
  fy3/1 -> Dot Product5/2

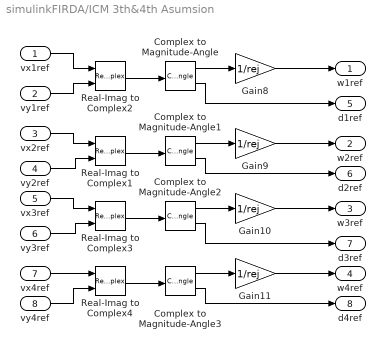
== system simulinkFIRDA/ICM 3th&4th Asumsion ==
  vx1ref : Inport
  vy1ref : Inport  Port=2
  vx2ref : Inport  Port=3
  vy2ref : Inport  Port=4
  vx3ref : Inport  Port=5
  vy3ref : Inport  Port=6
  vx4ref : Inport  Port=7
  vy4ref : Inport  Port=8
  Complex to Magnitude-Angle{,1..3} (4 alike) : ComplexToMagnitudeAngle
  Gain{8..11} (4 alike) : Gain  Gain=1/rej
  Real-Imag to Complex{1..4} (4 alike) : RealImagToComplex
  w1ref : Outport
  w2ref : Outport  Port=2
  w3ref : Outport  Port=3
  w4ref : Outport  Port=4
  d1ref : Outport  Port=5
  d2ref : Outport  Port=6
  d3ref : Outport  Port=7
  d4ref : Outport  Port=8
  wires:
  vx2ref/1 -> Real-Imag to Complex1/1
  vy1ref/1 -> Real-Imag to Complex2/2
  Gain8/1 -> w1ref/1
  Complex to Magnitude-Angle/2 -> d1ref/1
  Gain9/1 -> w2ref/1
  vy2ref/1 -> Real-Imag to Complex1/2
  Complex to Magnitude-Angle2/2 -> d3ref/1
  vx3ref/1 -> Real-Imag to Complex3/1
  vy4ref/1 -> Real-Imag to Complex4/2
  Complex to Magnitude-Angle3/1 -> Gain11/1
  Complex to Magnitude-Angle3/2 -> d4ref/1
  Real-Imag to Complex1/1 -> Complex to Magnitude-Angle1/1
  Complex to Magnitude-Angle1/2 -> d2ref/1
  vy3ref/1 -> Real-Imag to Complex3/2
  Complex to Magnitude-Angle/1 -> Gain8/1
  Gain11/1 -> w4ref/1
  vx1ref/1 -> Real-Imag to Complex2/1
  Gain10/1 -> w3ref/1
  vx4ref/1 -> Real-Imag to Complex4/1
  Real-Imag to Complex2/1 -> Complex to Magnitude-Angle/1
  Complex to Magnitude-Angle1/1 -> Gain9/1
  Real-Imag to Complex3/1 -> Complex to Magnitude-Angle2/1
  Complex to Magnitude-Angle2/1 -> Gain10/1
  Real-Imag to Complex4/1 -> Complex to Magnitude-Angle3/1

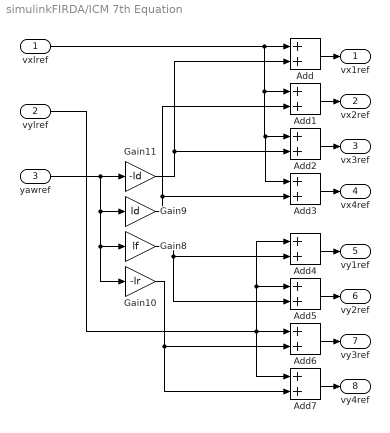
== system simulinkFIRDA/ICM 7th Equation ==
  vxlref : Inport
  vylref : Inport  Port=2
  yawref : Inport  Port=3
  Add{,1..7} (8 alike) : Sum
  Gain10 : Gain  Gain=-lr
  Gain11 : Gain  Gain=-ld
  Gain8 : Gain  Gain=lf
  Gain9 : Gain  Gain=ld
  vx1ref : Outport
  vx2ref : Outport  Port=2
  vx3ref : Outport  Port=3
  vx4ref : Outport  Port=4
  vy1ref : Outport  Port=5
  vy2ref : Outport  Port=6
  vy3ref : Outport  Port=7
  vy4ref : Outport  Port=8
  wires:
  Gain10/1 -> Add7/2, Add6/2
  Add1/1 -> vx2ref/1
  Gain8/1 -> Add4/2, Add5/2
  yawref/1 -> Gain9/1, Gain8/1, Gain10/1, Gain11/1
  vylref/1 -> Add7/1, Add6/1, Add5/1, Add4/1
  vxlref/1 -> Add3/1, Add2/1, Add1/1, Add/1
  Gain9/1 -> Add1/2, Add3/2
  Gain11/1 -> Add2/2, Add/2
  Add3/1 -> vx4ref/1
  Add/1 -> vx1ref/1
  Add5/1 -> vy2ref/1
  Add2/1 -> vx3ref/1
  Add4/1 -> vy1ref/1
  Add6/1 -> vy3ref/1
  Add7/1 -> vy4ref/1

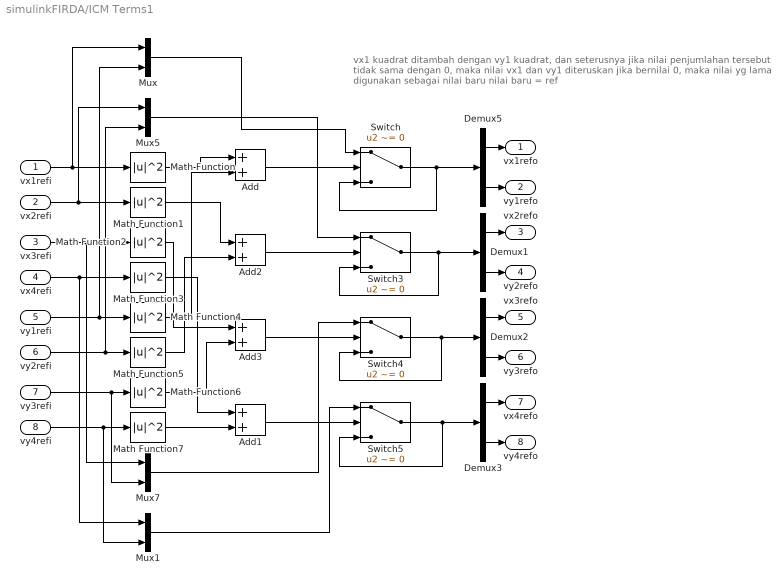
== system simulinkFIRDA/ICM Terms1 ==
  note: vx1 kuadrat ditambah dengan vy1 kuadrat, dan seterusnya
      | jika nilai penjumlahan tersebut tidak sama dengan 0, maka nilai vx1 dan vy1 diteruskan
      | jika bernilai 0, maka nilai yg lama digunakan sebagai nilai baru
      | nilai baru = ref
  vx1refi : Inport
  vx2refi : Inport  Port=2
  vx3refi : Inport  Port=3
  vx4refi : Inport  Port=4
  vy1refi : Inport  Port=5
  vy2refi : Inport  Port=6
  vy3refi : Inport  Port=7
  vy4refi : Inport  Port=8
  Add{,1..3} (4 alike) : Sum
  Demux{1..3,5} (4 alike) : Demux  Outputs=2
  Math Function{,1..7} (8 alike) : Math  Operator=magnitude^2  SignedPower=on  SaturateOnIntegerOverflow=on
  Mux{,1,5,7} (4 alike) : Mux  Inputs=2
  Switch{,3..5} (4 alike) : Switch  Criteria=u2 ~= 0
  vx1refo : Outport
  vy1refo : Outport  Port=2
  vx2refo : Outport  Port=3
  vy2refo : Outport  Port=4
  vx3refo : Outport  Port=5
  vy3refo : Outport  Port=6
  vx4refo : Outport  Port=7
  vy4refo : Outport  Port=8
  wires:
  Add2/1 -> Switch3/2
  Switch3/1 -> Switch3/3, Demux1/1
  Math Function3/1 -> Add1/1
  Demux3/2 -> vy4refo/1
  Demux5/1 -> vx1refo/1
  Demux2/1 -> vx3refo/1
  Demux5/2 -> vy1refo/1
  Demux2/2 -> vy3refo/1
  Demux3/1 -> vx4refo/1
  Math Function5/1 -> Add2/2
  vx3refi/1 -> Mux7/1, Math Function2/1
  Switch4/1 -> Switch4/3, Demux2/1
  vx2refi/1 -> Math Function1/1, Mux5/1
  Math Function6/1 -> Add3/2
  vy4refi/1 -> Mux1/2, Math Function7/1
  Math Function/1 -> Add/1
  Mux5/1 -> Switch3/1
  Add/1 -> Switch/2
  Mux7/1 -> Switch4/1
  Add3/1 -> Switch4/2
  Switch5/1 -> Switch5/3, Demux3/1
  Math Function2/1 -> Add3/1
  vx4refi/1 -> Mux1/1, Math Function3/1
  vy3refi/1 -> Mux7/2, Math Function6/1
  vy2refi/1 -> Mux5/2, Math Function5/1
  Math Function1/1 -> Add2/1
  Switch/1 -> Switch/3, Demux5/1
  vx1refi/1 -> Mux/1, Math Function/1
  Math Function4/1 -> Add/2
  vy1refi/1 -> Mux/2, Math Function4/1
  Mux/1 -> Switch/1
  Math Function7/1 -> Add1/2
  Add1/1 -> Switch5/2
  Demux1/1 -> vx2refo/1
  Demux1/2 -> vy2refo/1
  ? -> ?
  Mux1/1 -> Switch5/1

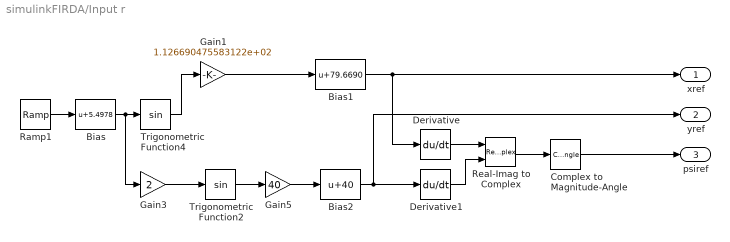
== system simulinkFIRDA/Input r ==
  Bias : Bias  Bias=5.4978
  Bias1 : Bias  Bias=79.6690
  Bias2 : Bias  Bias=40
  Complex to Magnitude-Angle : ComplexToMagnitudeAngle  Output=Angle
  Derivative : Derivative
  Derivative1 : Derivative
  Gain1 : Gain  Gain=1.126690475583122e+02
  Gain3 : Gain  Gain=2
  Gain5 : Gain  Gain=40
  Ramp1 : simulink/Sources/Ramp  slope=2*pi*Ts  start=0  InitialOutput=0  VectorParams1D=off
  Real-Imag to Complex : RealImagToComplex
  Trigonometric Function2 : Trigonometry
  Trigonometric Function4 : Trigonometry
  xref : Outport
  yref : Outport  Port=2
  "psiref " : Outport  Port=3
  wires:
  Trigonometric Function4/1 -> Gain1/1
  Gain5/1 -> Bias2/1
  Ramp1/1 -> Bias/1
  Bias/1 -> Gain3/1, Trigonometric Function4/1
  Gain1/1 -> Bias1/1
  Bias1/1 -> Derivative/1, xref/1
  Gain3/1 -> Trigonometric Function2/1
  Trigonometric Function2/1 -> Gain5/1
  Bias2/1 -> yref/1, Derivative1/1
  Derivative/1 -> Real-Imag to Complex/1
  Derivative1/1 -> Real-Imag to Complex/2
  Real-Imag to Complex/1 -> Complex to Magnitude-Angle/1
  Complex to Magnitude-Angle/1 -> "psiref "/1

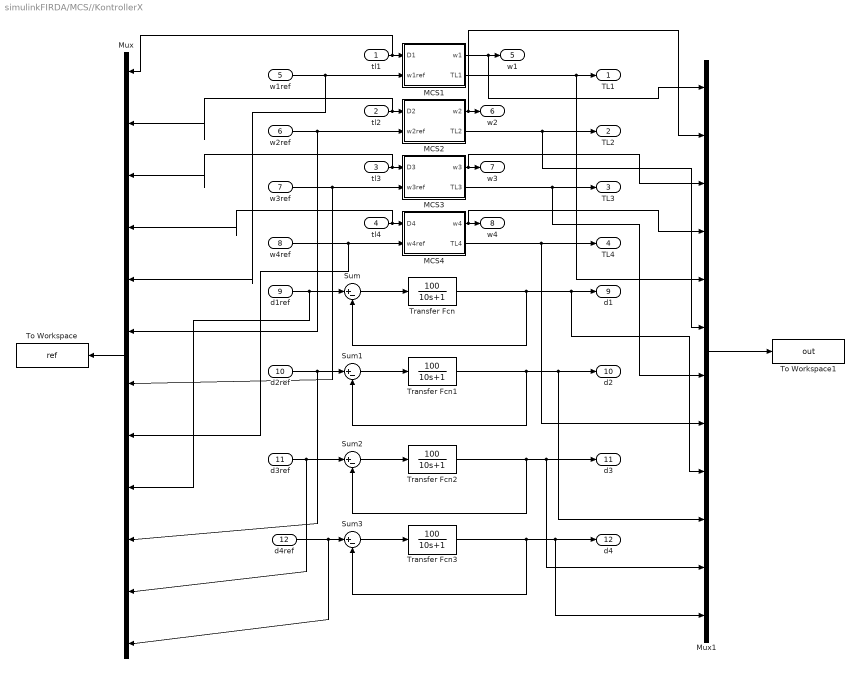
== system simulinkFIRDA/MCS//KontrollerX ==
  tl1 : Inport
  tl2 : Inport  Port=2
  tl3 : Inport  Port=3
  tl4 : Inport  Port=4
  w1ref : Inport  Port=5
  w2ref : Inport  Port=6
  w3ref : Inport  Port=7
  w4ref : Inport  Port=8
  d1ref : Inport  Port=9
  d2ref : Inport  Port=10
  d3ref : Inport  Port=11
  d4ref : Inport  Port=12
  MCS1 : Subsystem  mask(MCS){}
      mask help: Kontroller X
  MCS2 : Subsystem  mask(MCS){}
      mask help: Kontroller X
  MCS3 : Subsystem  mask(MCS){}
      mask help: Kontroller X
  MCS4 : Subsystem  mask(MCS){}
      mask help: Kontroller X
  Mux : Mux  Inputs=12
  Mux1 : Mux  Inputs=12
  Sum{,1..3} (4 alike) : Sum  Inputs=|+-
  To Workspace : ToWorkspace  VariableName=ref  SaveFormat=Timeseries  SampleTime=-1
  To Workspace1 : ToWorkspace  VariableName=out  SaveFormat=Timeseries  SampleTime=-1
  Transfer Fcn{,1..3} (4 alike) : TransferFcn  Numerator=[100]  Denominator=[10 1]
  TL1 : Outport
  TL2 : Outport  Port=2
  TL3 : Outport  Port=3
  TL4 : Outport  Port=4
  w1 : Outport  Port=5
  w2 : Outport  Port=6
  w3 : Outport  Port=7
  w4 : Outport  Port=8
  d1 : Outport  Port=9
  d2 : Outport  Port=10
  d3 : Outport  Port=11
  d4 : Outport  Port=12
  wires:
  MCS1/2(TL1) -> Mux1/5, TL1/1
  MCS2/2(TL2) -> Mux1/6, TL2/1
  MCS3/2(TL3) -> Mux1/7, TL3/1
  MCS4/2(TL4) -> Mux1/8, TL4/1
  tl2/1 -> Mux/2, MCS2/1(D2)
  w4ref/1 -> Mux/8, MCS4/2(w4ref)
  tl1/1 -> Mux/1, MCS1/1(D1)
  tl4/1 -> Mux/4, MCS4/1(D4)
  w3ref/1 -> Mux/7, MCS3/2(w3ref)
  tl3/1 -> Mux/3, MCS3/1(D3)
  w2ref/1 -> Mux/6, MCS2/2(w2ref)
  MCS2/1(w2) -> Mux1/2, w2/1
  MCS3/1(w3) -> Mux1/3, w3/1
  MCS1/1(w1) -> Mux1/1, w1/1
  MCS4/1(w4) -> Mux1/4, w4/1
  Sum/1 -> Transfer Fcn/1
  d1ref/1 -> Mux/9, Sum/1
  Transfer Fcn/1 -> Sum/2, Mux1/9, d1/1
  d2ref/1 -> Mux/10, Sum1/1
  Sum1/1 -> Transfer Fcn1/1
  Transfer Fcn1/1 -> Mux1/10, d2/1, Sum1/2
  d3ref/1 -> Mux/11, Sum2/1
  Sum3/1 -> Transfer Fcn3/1
  Transfer Fcn3/1 -> Mux1/12, d4/1, Sum3/2
  d4ref/1 -> Mux/12, Sum3/1
  Sum2/1 -> Transfer Fcn2/1
  Transfer Fcn2/1 -> Sum2/2, Mux1/11, d3/1
  w1ref/1 -> Mux/5, MCS1/2(w1ref)
  Mux/1 -> To Workspace/1
  Mux1/1 -> To Workspace1/1

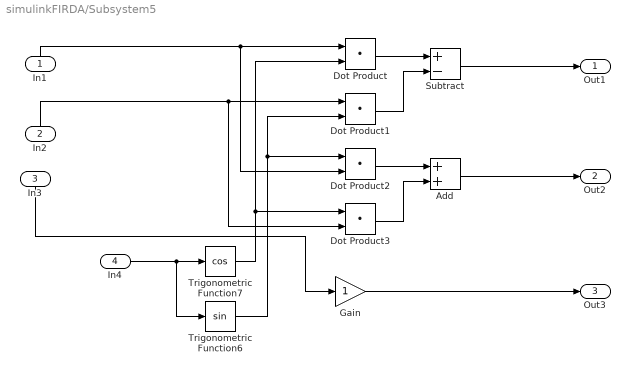
== system simulinkFIRDA/Subsystem5 ==
  In1 : Inport
  In2 : Inport  Port=2
  In3 : Inport  Port=3
  In4 : Inport  Port=4
  Add : Sum
  Dot Product{,1..3} (4 alike) : DotProduct  InputSameDT=on  OutDataTypeStr=Inherit: Inherit via internal rule
  Gain : Gain
  Subtract : Sum  Inputs=+-
  Trigonometric Function6 : Trigonometry
  Trigonometric Function7 : Trigonometry  Operator=cos
  Out1 : Outport
  Out2 : Outport  Port=2
  Out3 : Outport  Port=3
  wires:
  Gain/1 -> Out3/1
  Dot Product1/1 -> Subtract/2
  Subtract/1 -> Out1/1
  Dot Product2/1 -> Add/1
  In3/1 -> Gain/1
  In1/1 -> Dot Product2/2, Dot Product/1
  In2/1 -> Dot Product3/2, Dot Product1/1
  Dot Product3/1 -> Add/2
  In4/1 -> Trigonometric Function6/1, Trigonometric Function7/1
  Trigonometric Function7/1 -> Dot Product3/1, Dot Product/2
  Trigonometric Function6/1 -> Dot Product2/1, Dot Product1/2
  Add/1 -> Out2/1
  Dot Product/1 -> Subtract/1

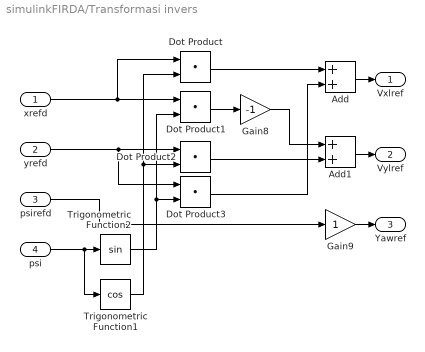
== system simulinkFIRDA/Transformasi invers  ==
  xrefd : Inport
  yrefd : Inport  Port=2
  psirefd : Inport  Port=3
  psi : Inport  Port=4
  Add : Sum
  Add1 : Sum
  Dot Product{,1..3} (4 alike) : DotProduct  InputSameDT=on  OutDataTypeStr=Inherit: Inherit via internal rule
  Gain8 : Gain  Gain=-1
  Gain9 : Gain
  Trigonometric Function1 : Trigonometry  Operator=cos
  Trigonometric Function2 : Trigonometry
  Vxlref : Outport
  Vylref : Outport  Port=2
  Yawref : Outport  Port=3
  wires:
  Trigonometric Function2/1 -> Dot Product1/2, Dot Product3/2
  Gain9/1 -> Yawref/1
  Add1/1 -> Vylref/1
  Dot Product3/1 -> Add/2
  psirefd/1 -> Gain9/1
  Dot Product1/1 -> Gain8/1
  Add/1 -> Vxlref/1
  xrefd/1 -> Dot Product1/1, Dot Product/1
  Dot Product2/1 -> Add1/2
  psi/1 -> Trigonometric Function1/1, Trigonometric Function2/1
  yrefd/1 -> Dot Product2/1, Dot Product3/1
  Trigonometric Function1/1 -> Dot Product2/2, Dot Product/2
  Dot Product/1 -> Add/1
  Gain8/1 -> Add1/1

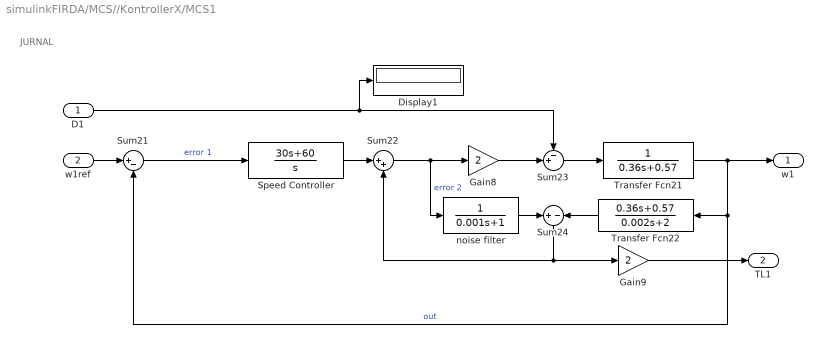
== system simulinkFIRDA/MCS//KontrollerX/MCS1 ==
  note: JURNAL
  D1 : Inport
  w1ref : Inport  Port=2
  Display1 : Display
  Gain8 : Gain  Gain=2
  Gain9 : Gain  Gain=2
  Speed Controller : TransferFcn  Numerator=[30 60]  Denominator=[1 0]
  Sum21 : Sum  Inputs=|+-
  Sum22 : Sum  Inputs=|++
  Sum23 : Sum  Inputs=-+|
  Sum24 : Sum  Inputs=+-
  Transfer Fcn21 : TransferFcn  Denominator=[0.36 0.57]
  Transfer Fcn22 : TransferFcn  Numerator=[0.36 0.57]  Denominator=[0.002 2]
  noise filter : TransferFcn  Denominator=[0.001 1]
  w1 : Outport
  TL1 : Outport  Port=2
  wires:
  Sum22/1 -> noise filter/1, Gain8/1  "error 2"
  Gain8/1 -> Sum23/2
  Transfer Fcn22/1 -> Sum24/2
  Speed Controller/1 -> Sum22/1
  noise filter/1 -> Sum24/1
  Sum24/1 -> Sum22/2, Gain9/1
  Sum21/1 -> Speed Controller/1  "error 1"
  Sum23/1 -> Transfer Fcn21/1
  Transfer Fcn21/1 -> w1/1, Sum21/2, Transfer Fcn22/1  "out"
  D1/1 -> Display1/1, Sum23/1
  Gain9/1 -> TL1/1
  w1ref/1 -> Sum21/1

== system simulinkFIRDA/MCS//KontrollerX/MCS2 ==
  D2 : Inport
  w2ref : Inport  Port=2
  Gain8 : Gain  Gain=2
  Gain9 : Gain  Gain=2
  Sum21 : Sum  Inputs=|+-
  Sum22 : Sum  Inputs=|++
  Sum23 : Sum  Inputs=-+|
  Sum24 : Sum  Inputs=+-
  Transfer Fcn19 : TransferFcn  Numerator=[30 60]  Denominator=[1 0]
  Transfer Fcn20 : TransferFcn  Denominator=[0.001 1]
  Transfer Fcn21 : TransferFcn  Denominator=[0.36 0.57]
  Transfer Fcn22 : TransferFcn  Numerator=[0.36 0.57]  Denominator=[0.002 2]
  w2 : Outport
  TL2 : Outport  Port=2
  wires:
  Sum22/1 -> Transfer Fcn20/1, Gain8/1
  Gain8/1 -> Sum23/2
  Transfer Fcn22/1 -> Sum24/2
  Transfer Fcn19/1 -> Sum22/1
  Transfer Fcn20/1 -> Sum24/1
  Sum24/1 -> Sum22/2, Gain9/1
  Sum21/1 -> Transfer Fcn19/1
  Sum23/1 -> Transfer Fcn21/1
  Transfer Fcn21/1 -> w2/1, Sum21/2, Transfer Fcn22/1
  D2/1 -> Sum23/1
  w2ref/1 -> Sum21/1
  Gain9/1 -> TL2/1

== system simulinkFIRDA/MCS//KontrollerX/MCS3 ==
  D3 : Inport
  w3ref : Inport  Port=2
  Gain8 : Gain  Gain=2
  Gain9 : Gain  Gain=2
  Sum21 : Sum  Inputs=|+-
  Sum22 : Sum  Inputs=|++
  Sum23 : Sum  Inputs=-+|
  Sum24 : Sum  Inputs=+-
  Transfer Fcn19 : TransferFcn  Numerator=[30 60]  Denominator=[1 0]
  Transfer Fcn20 : TransferFcn  Denominator=[0.001 1]
  Transfer Fcn21 : TransferFcn  Denominator=[0.36 0.57]
  Transfer Fcn22 : TransferFcn  Numerator=[0.36 0.57]  Denominator=[0.002 2]
  w3 : Outport
  TL3 : Outport  Port=2
  wires:
  Sum22/1 -> Transfer Fcn20/1, Gain8/1
  Gain8/1 -> Sum23/2
  Transfer Fcn22/1 -> Sum24/2
  Transfer Fcn19/1 -> Sum22/1
  Transfer Fcn20/1 -> Sum24/1
  Sum24/1 -> Sum22/2, Gain9/1
  Sum21/1 -> Transfer Fcn19/1
  Sum23/1 -> Transfer Fcn21/1
  Transfer Fcn21/1 -> w3/1, Sum21/2, Transfer Fcn22/1
  D3/1 -> Sum23/1
  w3ref/1 -> Sum21/1
  Gain9/1 -> TL3/1

== system simulinkFIRDA/MCS//KontrollerX/MCS4 ==
  D4 : Inport
  w4ref : Inport  Port=2
  Gain8 : Gain  Gain=2
  Gain9 : Gain  Gain=2
  Sum21 : Sum  Inputs=|+-
  Sum22 : Sum  Inputs=|++
  Sum23 : Sum  Inputs=-+|
  Sum24 : Sum  Inputs=+-
  Transfer Fcn19 : TransferFcn  Numerator=[30 60]  Denominator=[1 0]
  Transfer Fcn20 : TransferFcn  Denominator=[0.001 1]
  Transfer Fcn21 : TransferFcn  Denominator=[0.36 0.57]
  Transfer Fcn22 : TransferFcn  Numerator=[0.36 0.57]  Denominator=[0.002 2]
  w4 : Outport
  TL4 : Outport  Port=2
  wires:
  Sum22/1 -> Transfer Fcn20/1, Gain8/1
  Gain8/1 -> Sum23/2
  Transfer Fcn22/1 -> Sum24/2
  Transfer Fcn19/1 -> Sum22/1
  Transfer Fcn20/1 -> Sum24/1
  Sum24/1 -> Sum22/2, Gain9/1
  Sum21/1 -> Transfer Fcn19/1
  Sum23/1 -> Transfer Fcn21/1
  Transfer Fcn21/1 -> w4/1, Sum21/2, Transfer Fcn22/1
  D4/1 -> Sum23/1
  w4ref/1 -> Sum21/1
  Gain9/1 -> TL4/1

== matlab function simulinkFIRDA/MATLAB Function ==
  data: vxl input; vyl input; yaw input; vxld input; V1rm output; V2rm output; V3rm output; V4rm output; vyld input; yawd input; Ts parameter
function [V1rm,V2rm,V3rm,V4rm]= fcn( vxl,vyl,yaw,vxld,vyld,yawd, Ts)


 
% Ts = 0.01;                            % sampling time
% Np = 10;
% Nc =2;
%runTime =100;                          % stop time
nIteration = runTime/Ts;                % iteration
fdyn=zeros(1,nIteration);
X=zeros(3,nIteration);
u=zeros(4,nIteration);
Xdot=zeros(3,nIteration);

lmd=zeros(1,nIteration);
lmddot=zeros(1,nIteration);
Hu= zeros(1,nIteration);
Hx=zeros(1,nIteration);
P=zeros(1,nIteration);
F=zeros(1,nIteration);
dF=zeros(1,nIteration);
 
 % State Vector (X)& Control Vector (u)
 X(:,1) = [vxl;vyl;yaw];
 u(:,1) = [V1rm,V2rm,V3rm,V4rm]';
 Xdot(:,1) = [vxld;vyld;yawd];
 %X(0)=0;                                 % Initial condition
%fdyn(X,u)=Xdot;                         % Vehicle dynamic

% Set the constraints for manipulated variables.
Vjmax = 80;                             % Maximum speed of each tire 80 km/h
Vjmin = 0;                              % Minimum speed of each tire 0 m/s^2
Vmax = 100;                             % Maximum speed of vehicle 100 km/h
Vmin = 0;                               % Minimum speed of vehicle 0 m/s^2
Betamin = -1.5708;                      % Minimum side slip angle of vehicle -90 deg 
Betamax = 1.5708;                       % Maximum side slip angle of vehicle 90 deg
% * |xc| contains the state constraints.
% * |uc| contains the input constraint.
xc=[Vmin Vmax Betamin Betamax];
uc= [Vjmin Vjmax];
C=[xc;uc];

for k=1:nIteration
  for  j=1:4
    
    X(k+1)= X(k)+ (Ts*fdyn(X(k),u(k)));
    
    % Performance Index
    LcostfcnQ = symsum((X(k+1)-Xref(k+1)).' *Q * symsum(X(k+1,k)-Xref(k+1)), k, 0, Np);
    LcostfcnR = symsum((u(j,k+1,k)-u(j,k)).' *R * symsum(u(j,k+1,k)-u(j,k)), k, 0, Nc);
    J = 0.5*(LcostfcnQ+symsum((LcostfcnR),k,1,4)); 
    
    % Hamiltonian
    % lmd = costate
    % nu = Lagrange multipliers
    H = J+ (0.5*((lmd.' *fdyn)+(nu.'*C)));
    
    % Euler-Lagrange equations are obtained as the necessary conditions for the 
    % optimal solution. 
    Xdot(k)=fdyn(X(k),u(k));
    X(k)=X(0);
    lmddot(k) = Hx(X(k),lmd(k),u(k),nu(k))';    % d(H(X(k),lmd(k),u(k),nu(k)))'/dx
    Hu(X(k),lmd(k),u(k),nu(k)) = 0;             % d(H(X(k),lmd(k),u(k),nu(k)))/du
    C(X(k),u(k))=0;
    
    % Dividing the horizon into step, it is discretized the 
    % optimal control problem on the -axis with the forward difference as follows:
    for i=0:Np-1
    tau = k/Np;
    X(i+1,k)=X(i,k)+ (tau*fdyn(X(i,k),u(i,k)));
    X(0)=X(k);
    lmd(i,k)=lmd(i+1,k)+(tau*Hx(X(i,k),lmd(i+1,k),u(i,k),nu(i,k))');
    Hu(X(i,k),lmd(i+1,k),u(i,k),nu(i,k)) = 0;
    C(X(i,k),u(i,k))=0;
    
    % define a vector of the input and multipliers as :
    u(k) = [u(i)' nu(i)'];
    P(0)=u(i);
    
    F(X(0),u(0),0)=0;
    F(X(k),u(k),k)=[Hu(X(i,k),lmd(i+1,k),u(i,k),nu(i,k));C(X(i,k),u(i,k))];
    
    dF(X(k),u(k),k)=-As* F(X(k),u(k),k);
    
    % 1st Algorithm
    du=FDGMRES(u,X,Xdot,k,udot_hat,h,kmax);
    
    % 2nd Algorithm
    
    
    % U optimal :
    
    
   
    end
  end
end

== matlab function simulinkFIRDA/EVloop1&2(3)-(6)1/MATLAB Function1 ==
  data: Nx input; Ny input; m input; g input; h input; ld input; lf input; lr input; kro input; kfo input; fz1 output; fz2 output; fz3 output; fz4 output
function [fz1,fz2,fz3,fz4]  = invers(Nx,Ny,m,g,h,ld,lf,lr,kro,kfo)

N=[Nx Ny]';
Fzs=(m*g/2)*[lr/(lf+lr) lr/(lf+lr) lf/(lf+lr) lf/(lf+lr)]';
G=(h/(2*ld))*[ld/(lf+lr) ld/(lf+lr) -ld/(lf+lr) -ld/(lf+lr);
    kfo/(kfo+kro) -kfo/(kfo+kro) kro/(kfo+kro) -kro/(kfo+kro)]';
miu=eye(4,4)+(G*N);
fz=miu\Fzs;
fz1=fz(1,1);
fz2=fz(2,1);
fz3=fz(3,1);
fz4=fz(4,1);

== matlab function simulinkFIRDA/Menghtiung epsi dlm [-pi,pi] ==
  data: th2 input; th1 input; d output
function d = angdiff(th2, th1)
  
    switch nargin
        case 1
            if length(th1) == 2
                d = th1(1) - th1(2);
            else
                d = th1;
            end
        case 2
            if length(th1) > 1 && length(th2) > 1
                % if both arguments are vectors, they must be the same
                assert(all(size(th1) == size(th2)), 'SMTB:angdiff:badarg', 'vectors must be same shape');
            end
            % th1 or th2 could be scalar
            d = th1 - th2;
    end
    
    % wrap the result into the interval [-pi pi)
    d = mod(d+pi, 2*pi) - pi;
end

% Simplistic version of the code, easy to see what it does, but slow...
%
% for very negative angles keep adding 2pi
%     while true
%         k = find(d < -pi);
%         if isempty(k)
%             break;
%         end
%         d(k) = d(k) + 2*pi;
%     end
% 
%     % for very positive angles keep subtracting 2pi
%     while true
%         k = find(d > pi);
%         if isempty(k)
%             break;
%         end
%         d(k) = d(k) - 2*pi;
%     end
